simulink model "background_subtraction"  (R2013b)
settings: Solver=ode45  StartTime=0.0  StopTime=10.0  RelTol=1e-3
settings Model: Creator=Holly  LastModifiedBy=Holly

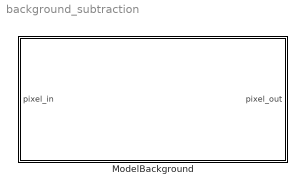
== system background_subtraction ==
  "ModelBackground " : Stateflow chart  TreatAsAtomicUnit=on

== stateflow chart background_subtraction/ModelBackground  ==
  state i = 0;
    j = 0;
    i_max = total pixels/num cores;
    j_max = num images;
  state i = 0;
    j = 0;
  state i = 0;
    j = 0;
  state i = 0;
  state Load image
    J += 1;
  state I = 0;
    j = 0;
  state Load2 image
    J += 1;
  state Load1 image
    J += 1;
  state Load3 image
    J += 1;
  state Calculate a;
    Calculate b;
    i++;
  state Read in pixel i
    i += 1;
  state Read2 in pixel i
    i += 1;
  state Read1 in pixel i
    i += 1;
  state Read3 in pixel i
    i += 1;
  state totalR += P[i].r
    totalG += P[i].g
    totalB += P[i].b
  state Done training
  state Calculate
    standard
    deviation
  state Calculate
    alpha
  state Calculate
    CD
  state avgR = totalR/n
    avgG = totalG/n
    avgB = totalB/n
  (default) -> i = 0; [order 1]
  i = 0; -> Load image
  totalR += P[i].r -> Load image [order 2] : i = i_max
      | && j < j_max
  Calculate -> i = 0; [order 3]
  (default) -> i = 0; [order 2] : if i = i+max
      | && j = j_max
  Calculate -> i = 0; [order 2]
  avgR = totalR/n -> I = 0;
  i = 0; -> Calculate a;
  i = 0; -> Load2 image
  i = 0; -> Load3 image
  Load image -> Read in pixel i
  I = 0; -> Load1 image
  Calculate -> Load2 image [order 3] : i = i_max
      | && j < j_max
  Calculate -> Load1 image [order 2] : i = i_max
      | && j < j_max
  Calculate -> Load3 image [order 2] : i = i_max
      | && j < j_max
  totalR += P[i].r -> Read in pixel i [order 1] : i < i_max
  Calculate a; -> Calculate a; [order 1] : i < i_max
  Load2 image -> Read2 in pixel i
  Load1 image -> Read1 in pixel i
  Load3 image -> Read3 in pixel i
  Calculate a; -> Done training [order 2] : i = i_max
  Read in pixel i -> totalR += P[i].r
  Calculate -> Read3 in pixel i [order 1] : i < i_max
  Calculate -> Read2 in pixel i [order 1] : i < i_max
  Calculate -> Read1 in pixel i [order 1] : i < i_max
  Read2 in pixel i -> Calculate
  Read1 in pixel i -> Calculate
  Read3 in pixel i -> Calculate
  totalR += P[i].r -> avgR = totalR/n [order 3] : if i = i+max
      | && j = j_max
  data: pixel_in input; pixel_out output double
